simulink model "crazyflie"  (R2015b)
settings: Solver=FixedStepAuto  StartTime=0.0  StopTime=18  FixedStep=1/500  MinStep=1e-4  RelTol=1e-3
undefined symbols (not defined in the file): A, B, C, D
libraries: simulink x1
(part 2 of 3)

== system crazyflie/Off-board ILQR Position Controller/Subsystem2 ==
  Rollw : Inport
  Pitchw : Inport  Port=2
  Measured Yaw : Inport  Port=3
  Demux : Demux  Outputs=2
  MATLAB Function : MATLAB Function  TreatAsAtomicUnit=on
  Mux : Mux  Inputs=2
  Product : Product  Multiplication=Matrix(*)
  Rollb Error : Outport
  Pitchb Error : Outport  Port=2
  wires:
  Rollw/1 -> Mux/1
  Pitchw/1 -> Mux/2
  Product/1 -> Demux/1
  Demux/1 -> Rollb Error/1
  Demux/2 -> Pitchb Error/1
  Measured Yaw/1 -> MATLAB Function/1(yaw)
  MATLAB Function/1(R_m) -> Product/1
  Mux/1 -> Product/2  "Xw Error"

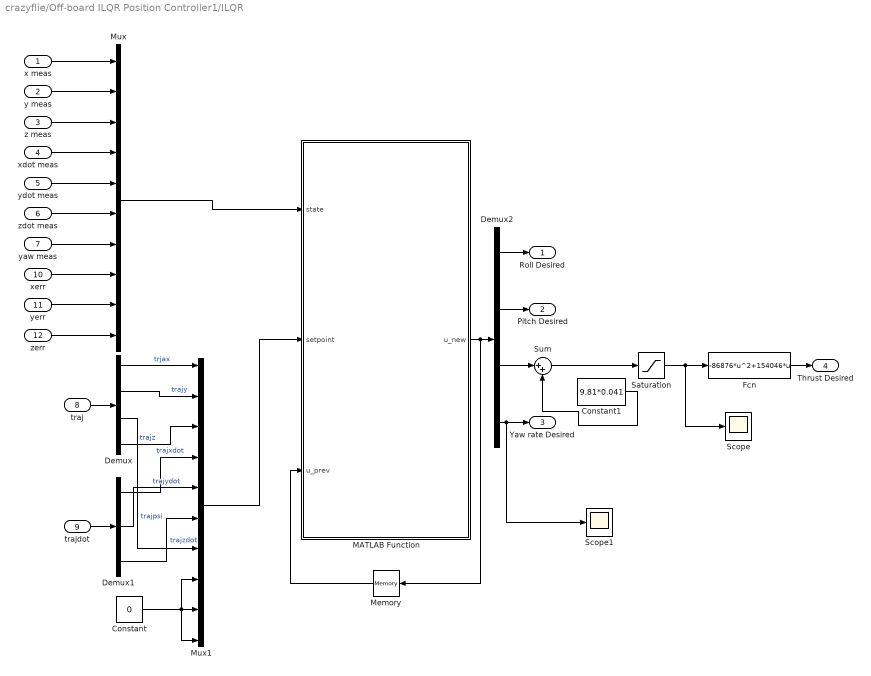
== system crazyflie/Off-board ILQR Position Controller1/ILQR ==
  x meas : Inport
  y meas : Inport  Port=2
  z meas : Inport  Port=3
  xdot meas : Inport  Port=4
  ydot meas : Inport  Port=5
  zdot meas : Inport  Port=6
  "yaw meas " : Inport  Port=7
  traj : Inport  Port=8
  trajdot : Inport  Port=9
  xerr : Inport  Port=10
  yerr : Inport  Port=11
  zerr : Inport  Port=12
  Constant : Constant  Value=0
  Constant1 : Constant  Value=9.81*0.041
  Demux : Demux
  Demux1 : Demux  Outputs=3
  Demux2 : Demux
  Fcn : Fcn  Expr=-86876*u^2+154046*u
  MATLAB Function : MATLAB Function  TreatAsAtomicUnit=on
  Memory : Memory  X0=[0 0 0 0]'
  Mux : Mux  Inputs=10
  Mux1 : Mux  Inputs=10
  Saturation : Saturate  UpperLimit=0.65  LowerLimit=0
  Scope : Scope
  Scope1 : Scope
  Sum : Sum  Inputs=|++
  Roll Desired : Outport
  Pitch Desired : Outport  Port=2
  Yaw rate Desired : Outport  Port=3
  Thrust Desired : Outport  Port=4
  wires:
  x meas/1 -> Mux/1
  y meas/1 -> Mux/2
  Fcn/1 -> Thrust Desired/1
  z meas/1 -> Mux/3
  ydot meas/1 -> Mux/5
  zdot meas/1 -> Mux/6
  "yaw meas "/1 -> Mux/7
  xdot meas/1 -> Mux/4
  Sum/1 -> Saturation/1
  Constant1/1 -> Sum/2
  traj/1 -> Demux/1
  trajdot/1 -> Demux1/1
  Mux/1 -> MATLAB Function/1(state)
  Mux1/1 -> MATLAB Function/2(setpoint)
  Demux/1 -> Mux1/1  "trjax"
  Demux/2 -> Mux1/2  "trajy"
  Demux/4 -> Mux1/3  "trajz"
  Demux1/1 -> Mux1/4  "trajxdot"
  Demux1/2 -> Mux1/5  "trajydot"
  Demux1/3 -> Mux1/6  "trajzdot"
  Demux/3 -> Mux1/7  "trajpsi"
  MATLAB Function/1(u_new) -> Demux2/1, Memory/1
  Memory/1 -> MATLAB Function/3(u_prev)
  Demux2/1 -> Roll Desired/1
  Demux2/2 -> Pitch Desired/1
  Demux2/4 -> Yaw rate Desired/1, Scope1/1
  Demux2/3 -> Sum/1
  Saturation/1 -> Scope/1, Fcn/1
  Constant/1 -> Mux1/10, Mux1/8, Mux1/9
  xerr/1 -> Mux/8
  yerr/1 -> Mux/9
  zerr/1 -> Mux/10

== system crazyflie/Off-board ILQR Position Controller1/Subsystem2 ==
  Rollw : Inport
  Pitchw : Inport  Port=2
  Measured Yaw : Inport  Port=3
  Demux : Demux  Outputs=2
  MATLAB Function : MATLAB Function  TreatAsAtomicUnit=on
  Mux : Mux  Inputs=2
  Product : Product  Multiplication=Matrix(*)
  Rollb Error : Outport
  Pitchb Error : Outport  Port=2
  wires:
  Rollw/1 -> Mux/1
  Pitchw/1 -> Mux/2
  Product/1 -> Demux/1
  Demux/1 -> Rollb Error/1
  Demux/2 -> Pitchb Error/1
  Measured Yaw/1 -> MATLAB Function/1(yaw)
  MATLAB Function/1(R_m) -> Product/1
  Mux/1 -> Product/2  "Xw Error"

== system crazyflie/Off-board LQR Position Controller /LQR ==
  xe : Inport
  ye : Inport  Port=2
  ze : Inport  Port=3
  xdote : Inport  Port=4
  ydote : Inport  Port=5
  zdote : Inport  Port=6
  "yawe " : Inport  Port=7
  xe int : Inport  Port=8
  ye int : Inport  Port=9
  ze int : Inport  Port=10
  Constant : Constant  Value="[5.60004970078151\t8.58620031779818e-15\t1.79188398034056e-13\t10.0569231021990\t1.51538658702357e-16\t6.75183288667297e-14\t-5.69346371635233e-16\t0.316227766016842\t1.15721882726472e-16\t7.37858743577978e-16;-4.45384218978841e-15\t5.60004970078150\t1.40244562919347e-12\t1.51538658702357e-16\t10.0569231021990\t2.52099816991567e-13\t-1.20831577789100e-16\t3.71448157568776e-15\t0.316227766016834\t6.21616501237700e-13;-1.24071227397705e-14\t1.04992513941598e-14\t316.738599971154\t1.66810943507647e-17\t6.22838406049332e-17\t511.246554592667\t-5.10238077464527e-16\t-2.21761716133426e-16\t9.39771534804335e-15\t0.316227766016796;-5.87842517815967e-15\t-1.61107236968454e-15\t-1.26223470684901e-13\t-5.80373467518077e-17\t-1.23171842802345e-17\t-2.10523704707751e-13\t3.16227766016838\t-1.11614612446732e-15\t2.11077368256129e-16\t-6.41049593874995e-15]"
  Constant1 : Constant  Value=9.81*0.041
  Demux : Demux
  Fcn : Fcn  Expr=-86876*u^2+154046*u
  Mux : Mux  Inputs=10
  Product : Product  Multiplication=Matrix(*)
  Saturation : Saturate  UpperLimit=0.65  LowerLimit=-0.041*9.81
  Sum : Sum  Inputs=|++
  Roll Desired : Outport
  Pitch Desired : Outport  Port=2
  Yaw rate Desired : Outport  Port=3
  Thrust Desired : Outport  Port=4
  wires:
  xe/1 -> Mux/1
  ye/1 -> Mux/2
  Demux/1 -> Roll Desired/1
  Demux/2 -> Pitch Desired/1
  Fcn/1 -> Thrust Desired/1
  ze/1 -> Mux/3
  ydote/1 -> Mux/5
  zdote/1 -> Mux/6
  Demux/3 -> Saturation/1
  Demux/4 -> Yaw rate Desired/1
  Mux/1 -> Product/2
  Product/1 -> Demux/1
  Constant/1 -> Product/1
  "yawe "/1 -> Mux/7
  xdote/1 -> Mux/4
  xe int/1 -> Mux/8
  ye int/1 -> Mux/9
  ze int/1 -> Mux/10
  Saturation/1 -> Sum/1
  Sum/1 -> Fcn/1
  Constant1/1 -> Sum/2

== system crazyflie/Off-board LQR Position Controller /Subsystem ==
  X : Inport
  Measured X : Inport  Port=2
  Y : Inport  Port=3
  Measured Y : Inport  Port=4
  Measured Yaw : Inport  Port=5
  Demux : Demux  Outputs=2
  MATLAB Function : MATLAB Function  TreatAsAtomicUnit=on
  Mux : Mux  Inputs=2
  Product : Product  Multiplication=Matrix(*)
  Sum : Sum  Inputs=|+-
  Sum1 : Sum  Inputs=|+-
  Xb Error : Outport
  Yb Error : Outport  Port=2
  wires:
  X/1 -> Sum/1
  Measured X/1 -> Sum/2
  Y/1 -> Sum1/1
  Measured Y/1 -> Sum1/2
  Sum/1 -> Mux/1
  Sum1/1 -> Mux/2
  Product/1 -> Demux/1
  Demux/1 -> Xb Error/1
  Demux/2 -> Yb Error/1
  Measured Yaw/1 -> MATLAB Function/1(yaw)
  MATLAB Function/1(R_m) -> Product/1
  Mux/1 -> Product/2  "Xw Error"

== system crazyflie/Off-board LQR Position Controller /Subsystem1 ==
  Xdot : Inport
  Measured Xdot : Inport  Port=2
  Ydot : Inport  Port=3
  Measured Ydot : Inport  Port=4
  Measured Yaw : Inport  Port=5
  Demux : Demux  Outputs=2
  MATLAB Function : MATLAB Function  TreatAsAtomicUnit=on
  Mux : Mux  Inputs=2
  Product : Product  Multiplication=Matrix(*)
  Sum : Sum  Inputs=|+-
  Sum1 : Sum  Inputs=|+-
  Xdotb Error : Outport
  Ydotb Error : Outport  Port=2
  wires:
  Xdot/1 -> Sum/1
  Measured Xdot/1 -> Sum/2
  Ydot/1 -> Sum1/1
  Measured Ydot/1 -> Sum1/2
  Sum/1 -> Mux/1
  Sum1/1 -> Mux/2
  Product/1 -> Demux/1
  Demux/1 -> Xdotb Error/1
  Demux/2 -> Ydotb Error/1
  Measured Yaw/1 -> MATLAB Function/1(yaw)
  MATLAB Function/1(R_m) -> Product/1
  Mux/1 -> Product/2  "Xw Error"

== system crazyflie/Off-board PID Position Controller/Subsystem ==
  X : Inport
  Measured X : Inport  Port=2
  Y : Inport  Port=3
  Measured Y : Inport  Port=4
  Measured Yaw : Inport  Port=5
  Demux : Demux  Outputs=2
  MATLAB Function : MATLAB Function  TreatAsAtomicUnit=on
  Mux : Mux  Inputs=2
  Product : Product  Multiplication=Matrix(*)
  Sum : Sum  Inputs=|+-
  Sum1 : Sum  Inputs=|+-
  Xb Error : Outport
  Yb Error : Outport  Port=2
  wires:
  X/1 -> Sum/1
  Measured X/1 -> Sum/2
  Y/1 -> Sum1/1
  Measured Y/1 -> Sum1/2
  Sum/1 -> Mux/1
  Sum1/1 -> Mux/2
  Product/1 -> Demux/1
  Demux/1 -> Xb Error/1
  Demux/2 -> Yb Error/1
  Measured Yaw/1 -> MATLAB Function/1(yaw)
  MATLAB Function/1(R_m) -> Product/1
  Mux/1 -> Product/2  "Xw Error"

== system crazyflie/Off-board PID Position Controller/X PID ==
  Xb Error : Inport
  Derivative : Derivative
  Integrator : Integrator
  Kd : Gain  Gain=10
  Ki : Gain  Gain=4
  Kp : Gain  Gain=18
  Saturation : Saturate  UpperLimit=.2  LowerLimit=-.2
  Sine Wave : Sin  Amplitude=0  SampleTime=0
  Sum : Sum  Inputs=|++
  Sum3 : Sum  Inputs=+++
  X PID : Outport
  wires:
  Xb Error/1 -> Derivative/1, Integrator/1, Kp/1
  Kp/1 -> Sum3/1
  Kd/1 -> Sum3/3
  Ki/1 -> Sum3/2
  Saturation/1 -> Ki/1
  Integrator/1 -> Saturation/1
  Derivative/1 -> Kd/1
  Sum/1 -> X PID/1
  Sine Wave/1 -> Sum/2
  Sum3/1 -> Sum/1

== system crazyflie/Off-board PID Position Controller/Y PID ==
  Yb Error : Inport
  Derivative : Derivative
  Integrator : Integrator
  Kd : Gain  Gain=10
  Ki : Gain  Gain=4
  Kp : Gain  Gain=18
  Saturation : Saturate  UpperLimit=.2  LowerLimit=-.2
  Sine Wave : Sin  Amplitude=0  SampleTime=0
  Sum : Sum  Inputs=|++
  Sum3 : Sum  Inputs=+++
  Y PID : Outport
  wires:
  Yb Error/1 -> Derivative/1, Integrator/1, Kp/1
  Kp/1 -> Sum3/1
  Kd/1 -> Sum3/3
  Ki/1 -> Sum3/2
  Saturation/1 -> Ki/1
  Integrator/1 -> Saturation/1
  Derivative/1 -> Kd/1
  Sum/1 -> Y PID/1
  Sine Wave/1 -> Sum/2
  Sum3/1 -> Sum/1

== system crazyflie/Off-board PID Position Controller/Yaw PID ==
  Yaw : Inport
  Measured Yaw : Inport  Port=2
  Derivative : Derivative
  Integrator : Integrator
  Kd : Gain
  Ki : Gain  Gain=0
  Kp : Gain  Gain=3
  Saturation : Saturate  UpperLimit=.2  LowerLimit=-.2
  Sine Wave : Sin  Amplitude=0  SampleTime=0
  Sum : Sum  Inputs=|++
  Sum2 : Sum  Inputs=|+-
  Sum3 : Sum  Inputs=+++
  Yaw PID : Outport
  wires:
  Yaw/1 -> Sum2/1
  Measured Yaw/1 -> Sum2/2
  Sum2/1 -> Derivative/1, Integrator/1, Kp/1
  Kp/1 -> Sum3/1
  Kd/1 -> Sum3/3
  Ki/1 -> Sum3/2
  Saturation/1 -> Ki/1
  Integrator/1 -> Saturation/1
  Derivative/1 -> Kd/1
  Sine Wave/1 -> Sum/2
  Sum3/1 -> Sum/1
  Sum/1 -> Yaw PID/1

== system crazyflie/Off-board PID Position Controller/Z PID ==
  Z : Inport
  Measured Z : Inport  Port=2
  Derivative : Derivative
  Integrator : Integrator
  Kd : Gain  Gain=40000
  Ki : Gain  Gain=10000
  Kp : Gain  Gain=50000
  PID Limit : Saturate  UpperLimit=25000  LowerLimit=-25000
  Saturation : Saturate  UpperLimit=10  LowerLimit=-10
  Sine Wave : Sin  Amplitude=0  SampleTime=0
  Sum : Sum  Inputs=|++
  Sum1 : Sum  Inputs=|++
  Sum2 : Sum  Inputs=|+-
  Sum3 : Sum  Inputs=+++
  Thrust Base : Constant  Value=36500
  Z PID : Outport
  wires:
  Sum2/1 -> Integrator/1, Derivative/1, Kp/1
  Kp/1 -> Sum3/1
  Kd/1 -> Sum3/3
  Ki/1 -> Sum3/2
  Saturation/1 -> Ki/1
  Thrust Base/1 -> Sum/2
  Sum3/1 -> PID Limit/1
  PID Limit/1 -> Sum/1
  Z/1 -> Sum2/1
  Measured Z/1 -> Sum2/2
  Integrator/1 -> Saturation/1
  Derivative/1 -> Kd/1
  Sum/1 -> Sum1/1
  Sum1/1 -> Z PID/1
  Sine Wave/1 -> Sum1/2

== system crazyflie/Off-board PID Position Controller1/Subsystem ==
  X : Inport
  Measured X : Inport  Port=2
  Y : Inport  Port=3
  Measured Y : Inport  Port=4
  Measured Yaw : Inport  Port=5
  Demux : Demux  Outputs=2
  MATLAB Function : MATLAB Function  TreatAsAtomicUnit=on
  Mux : Mux  Inputs=2
  Product : Product  Multiplication=Matrix(*)
  Sum : Sum  Inputs=|+-
  Sum1 : Sum  Inputs=|+-
  Xb Error : Outport
  Yb Error : Outport  Port=2
  wires:
  X/1 -> Sum/1
  Measured X/1 -> Sum/2
  Y/1 -> Sum1/1
  Measured Y/1 -> Sum1/2
  Sum/1 -> Mux/1
  Sum1/1 -> Mux/2
  Product/1 -> Demux/1
  Demux/1 -> Xb Error/1
  Demux/2 -> Yb Error/1
  Measured Yaw/1 -> MATLAB Function/1(yaw)
  MATLAB Function/1(R_m) -> Product/1
  Mux/1 -> Product/2  "Xw Error"

== system crazyflie/Off-board PID Position Controller1/X PID ==
  Xb Error : Inport
  Derivative : Derivative
  Integrator : Integrator
  Kd : Gain  Gain=10
  Ki : Gain  Gain=4
  Kp : Gain  Gain=18
  Saturation : Saturate  UpperLimit=.2  LowerLimit=-.2
  Sum3 : Sum  Inputs=+++
  X PID : Outport
  wires:
  Xb Error/1 -> Derivative/1, Integrator/1, Kp/1
  Kp/1 -> Sum3/1
  Kd/1 -> Sum3/3
  Sum3/1 -> X PID/1
  Ki/1 -> Sum3/2
  Saturation/1 -> Ki/1
  Integrator/1 -> Saturation/1
  Derivative/1 -> Kd/1

== system crazyflie/Off-board PID Position Controller1/Y PID ==
  Yb Error : Inport
  Derivative : Derivative
  Integrator : Integrator
  Kd : Gain  Gain=10
  Ki : Gain  Gain=4
  Kp : Gain  Gain=18
  Saturation : Saturate  UpperLimit=.2  LowerLimit=-.2
  Sum3 : Sum  Inputs=+++
  Y PID : Outport
  wires:
  Yb Error/1 -> Derivative/1, Integrator/1, Kp/1
  Kp/1 -> Sum3/1
  Kd/1 -> Sum3/3
  Sum3/1 -> Y PID/1
  Ki/1 -> Sum3/2
  Saturation/1 -> Ki/1
  Integrator/1 -> Saturation/1
  Derivative/1 -> Kd/1

== system crazyflie/Off-board PID Position Controller1/Yaw PID ==
  Yaw : Inport
  Measured Yaw : Inport  Port=2
  Derivative : Derivative
  Integrator : Integrator
  Kd : Gain
  Ki : Gain  Gain=0
  Kp : Gain  Gain=3
  Saturation : Saturate  UpperLimit=.2  LowerLimit=-.2
  Sum2 : Sum  Inputs=|+-
  Sum3 : Sum  Inputs=+++
  Yaw PID : Outport
  wires:
  Yaw/1 -> Sum2/1
  Measured Yaw/1 -> Sum2/2
  Sum2/1 -> Derivative/1, Integrator/1, Kp/1
  Kp/1 -> Sum3/1
  Kd/1 -> Sum3/3
  Sum3/1 -> Yaw PID/1
  Ki/1 -> Sum3/2
  Saturation/1 -> Ki/1
  Integrator/1 -> Saturation/1
  Derivative/1 -> Kd/1

== system crazyflie/Off-board PID Position Controller1/Z PID ==
  Z : Inport
  Measured Z : Inport  Port=2
  Derivative : Derivative
  Integrator : Integrator
  Kd : Gain  Gain=40000
  Ki : Gain  Gain=10000
  Kp : Gain  Gain=50000
  PID Limit : Saturate  UpperLimit=25000  LowerLimit=-25000
  Saturation : Saturate  UpperLimit=10  LowerLimit=-10
  Sum : Sum  Inputs=|++
  Sum2 : Sum  Inputs=|+-
  Sum3 : Sum  Inputs=+++
  Thrust Base : Constant  Value=35125.3
  Z PID : Outport
  wires:
  Sum2/1 -> Integrator/1, Derivative/1, Kp/1
  Kp/1 -> Sum3/1
  Kd/1 -> Sum3/3
  Ki/1 -> Sum3/2
  Saturation/1 -> Ki/1
  Thrust Base/1 -> Sum/2
  Sum/1 -> Z PID/1
  Sum3/1 -> PID Limit/1
  PID Limit/1 -> Sum/1
  Z/1 -> Sum2/1
  Measured Z/1 -> Sum2/2
  Integrator/1 -> Saturation/1
  Derivative/1 -> Kd/1

== system crazyflie/On-board Controller/Attitude Controller  ==
  Roll : Inport
  Pitch : Inport  Port=2
  Measured Roll : Inport  Port=3
  Measured Pitch : Inport  Port=4
  Pitch PID : Subsystem
  Roll PID : Subsystem
  Desired Roll : Outport
  "Desired Pitch " : Outport  Port=2
  wires:
  Pitch/1 -> Pitch PID/1(Pitch)
  Measured Pitch/1 -> Pitch PID/2(Measured Pitch)
  Pitch PID/1(Pitch PID) -> "Desired Pitch "/1
  Measured Roll/1 -> Roll PID/2(Measured Roll)
  Roll/1 -> Roll PID/1(Roll)
  Roll PID/1(Roll PID) -> Desired Roll/1

== system crazyflie/On-board Controller/Attitude Rate Controller ==
  Roll Rate : Inport
  Pitch Rate : Inport  Port=2
  Measured Roll Rate : Inport  Port=3
  Measured Pitch Rate : Inport  Port=4
  Pitch Rate PID : Subsystem
  Roll Rate PID : Subsystem
  Saturation : Saturate  UpperLimit=2^15  LowerLimit=-2^15
  Saturation1 : Saturate  UpperLimit=2^15  LowerLimit=-2^15
  Commanded Roll : Outport
  Commanded Pitch : Outport  Port=2
  wires:
  Roll Rate/1 -> Roll Rate PID/1(Roll Rate)
  Measured Roll Rate/1 -> Roll Rate PID/2(Measured Roll Rate)
  Pitch Rate/1 -> Pitch Rate PID/1(Pitch Ratel)
  Measured Pitch Rate/1 -> Pitch Rate PID/2(Measured Pitch Rate)
  Roll Rate PID/1(Roll Rate PID) -> Saturation/1
  Pitch Rate PID/1(Pitch Rate PID) -> Saturation1/1
  Saturation/1 -> Commanded Roll/1
  Saturation1/1 -> Commanded Pitch/1

== system crazyflie/On-board Controller/Mixer ==
  Roll : Inport
  Pitch : Inport  Port=2
  Yawrate : Inport  Port=3
  Thrust : Inport  Port=4
  Display : Display
  Gain : Gain  Gain=.5
  Gain1 : Gain  Gain=.5
  Saturation{,1..3} (4 alike) : Saturate  UpperLimit=2^16  LowerLimit=0
  Sum : Sum  Inputs=-+++
  Sum1 : Sum  Inputs=---+
  Sum2 : Sum  Inputs=+-++
  Sum3 : Sum  Inputs=++-+
  Motor 1 : Outport
  Motor 2 : Outport  Port=2
  Motor 3 : Outport  Port=3
  Motor 4 : Outport  Port=4
  wires:
  Roll/1 -> Gain/1
  Pitch/1 -> Gain1/1
  Yawrate/1 -> Sum1/3, Sum/3, Sum3/3, Sum2/3
  Thrust/1 -> Sum2/4, Sum3/4, Sum1/4, Sum/4
  Sum/1 -> Saturation/1
  Sum2/1 -> Saturation2/1
  Sum3/1 -> Saturation3/1
  Sum1/1 -> Saturation1/1
  Gain/1 -> Sum3/1, Sum2/1, Sum1/1, Sum/1
  Gain1/1 -> Sum3/2, Sum2/2, Sum1/2, Sum/2
  Saturation1/1 -> Motor 2/1
  Saturation2/1 -> Motor 3/1
  Saturation3/1 -> Motor 4/1
  Saturation/1 -> Display/1, Motor 1/1

== system crazyflie/On-board Controller/Yawrate Controller  ==
  Desired Yawrate : Inport
  Measured Yawrate : Inport  Port=2
  Yawrate PID : Subsystem
  Commanded Yawrate : Outport
  wires:
  Yawrate PID/1(Yawrate PID) -> Commanded Yawrate/1
  Desired Yawrate/1 -> Yawrate PID/1(Yawrate)
  Measured Yawrate/1 -> Yawrate PID/2(Measured Yawrate)

== system crazyflie/On-board Controller1/Attitude Controller  ==
  Roll : Inport
  Pitch : Inport  Port=2
  Measured Roll : Inport  Port=3
  Measured Pitch : Inport  Port=4
  Pitch PID : Subsystem
  Roll PID : Subsystem
  Desired Roll : Outport
  "Desired Pitch " : Outport  Port=2
  wires:
  Pitch/1 -> Pitch PID/1(Pitch)
  Measured Pitch/1 -> Pitch PID/2(Measured Pitch)
  Pitch PID/1(Pitch PID) -> "Desired Pitch "/1
  Measured Roll/1 -> Roll PID/2(Measured Roll)
  Roll/1 -> Roll PID/1(Roll)
  Roll PID/1(Roll PID) -> Desired Roll/1

== system crazyflie/On-board Controller1/Attitude Rate Controller ==
  Roll Rate : Inport
  Pitch Rate : Inport  Port=2
  Measured Roll Rate : Inport  Port=3
  Measured Pitch Rate : Inport  Port=4
  Pitch Rate PID : Subsystem
  Roll Rate PID : Subsystem
  Saturation : Saturate  UpperLimit=2^15  LowerLimit=-2^15
  Saturation1 : Saturate  UpperLimit=2^15  LowerLimit=-2^15
  Commanded Roll : Outport
  Commanded Pitch : Outport  Port=2
  wires:
  Roll Rate/1 -> Roll Rate PID/1(Roll Rate)
  Measured Roll Rate/1 -> Roll Rate PID/2(Measured Roll Rate)
  Pitch Rate/1 -> Pitch Rate PID/1(Pitch Ratel)
  Measured Pitch Rate/1 -> Pitch Rate PID/2(Measured Pitch Rate)
  Roll Rate PID/1(Roll Rate PID) -> Saturation/1
  Pitch Rate PID/1(Pitch Rate PID) -> Saturation1/1
  Saturation/1 -> Commanded Roll/1
  Saturation1/1 -> Commanded Pitch/1

== system crazyflie/On-board Controller1/Mixer ==
  Roll : Inport
  Pitch : Inport  Port=2
  Yawrate : Inport  Port=3
  Thrust : Inport  Port=4
  Display : Display
  Gain : Gain  Gain=.5
  Gain1 : Gain  Gain=.5
  Saturation{,1..3} (4 alike) : Saturate  UpperLimit=2^16  LowerLimit=0
  Sum : Sum  Inputs=-+++
  Sum1 : Sum  Inputs=---+
  Sum2 : Sum  Inputs=+-++
  Sum3 : Sum  Inputs=++-+
  Motor 1 : Outport
  Motor 2 : Outport  Port=2
  Motor 3 : Outport  Port=3
  Motor 4 : Outport  Port=4
  wires:
  Roll/1 -> Gain/1
  Pitch/1 -> Gain1/1
  Yawrate/1 -> Sum1/3, Sum/3, Sum3/3, Sum2/3
  Thrust/1 -> Sum2/4, Sum3/4, Sum1/4, Sum/4
  Sum/1 -> Saturation/1
  Sum2/1 -> Saturation2/1
  Sum3/1 -> Saturation3/1
  Sum1/1 -> Saturation1/1
  Gain/1 -> Sum3/1, Sum2/1, Sum1/1, Sum/1
  Gain1/1 -> Sum3/2, Sum2/2, Sum1/2, Sum/2
  Saturation1/1 -> Motor 2/1
  Saturation2/1 -> Motor 3/1
  Saturation3/1 -> Motor 4/1
  Saturation/1 -> Display/1, Motor 1/1

== system crazyflie/On-board Controller1/Yawrate Controller  ==
  Desired Yawrate : Inport
  Measured Yawrate : Inport  Port=2
  Yawrate PID : Subsystem
  Commanded Yawrate : Outport
  wires:
  Yawrate PID/1(Yawrate PID) -> Commanded Yawrate/1
  Desired Yawrate/1 -> Yawrate PID/1(Yawrate)
  Measured Yawrate/1 -> Yawrate PID/2(Measured Yawrate)

== system crazyflie/On-board Controller2/Attitude Controller  ==
  Roll : Inport
  Pitch : Inport  Port=2
  Measured Roll : Inport  Port=3
  Measured Pitch : Inport  Port=4
  Pitch PID : Subsystem
  Roll PID : Subsystem
  Desired Roll : Outport
  "Desired Pitch " : Outport  Port=2
  wires:
  Pitch/1 -> Pitch PID/1(Pitch)
  Measured Pitch/1 -> Pitch PID/2(Measured Pitch)
  Pitch PID/1(Pitch PID) -> "Desired Pitch "/1
  Measured Roll/1 -> Roll PID/2(Measured Roll)
  Roll/1 -> Roll PID/1(Roll)
  Roll PID/1(Roll PID) -> Desired Roll/1

== system crazyflie/On-board Controller2/Attitude Rate Controller ==
  Roll Rate : Inport
  Pitch Rate : Inport  Port=2
  Measured Roll Rate : Inport  Port=3
  Measured Pitch Rate : Inport  Port=4
  Pitch Rate PID : Subsystem
  Roll Rate PID : Subsystem
  Saturation : Saturate  UpperLimit=2^15  LowerLimit=-2^15
  Saturation1 : Saturate  UpperLimit=2^15  LowerLimit=-2^15
  Commanded Roll : Outport
  Commanded Pitch : Outport  Port=2
  wires:
  Roll Rate/1 -> Roll Rate PID/1(Roll Rate)
  Measured Roll Rate/1 -> Roll Rate PID/2(Measured Roll Rate)
  Pitch Rate/1 -> Pitch Rate PID/1(Pitch Ratel)
  Measured Pitch Rate/1 -> Pitch Rate PID/2(Measured Pitch Rate)
  Roll Rate PID/1(Roll Rate PID) -> Saturation/1
  Pitch Rate PID/1(Pitch Rate PID) -> Saturation1/1
  Saturation/1 -> Commanded Roll/1
  Saturation1/1 -> Commanded Pitch/1

== system crazyflie/On-board Controller2/Mixer ==
  Roll : Inport
  Pitch : Inport  Port=2
  Yawrate : Inport  Port=3
  Thrust : Inport  Port=4
  Display : Display
  Gain : Gain  Gain=.5
  Gain1 : Gain  Gain=.5
  Saturation{,1..3} (4 alike) : Saturate  UpperLimit=2^16  LowerLimit=0
  Sum : Sum  Inputs=-+++
  Sum1 : Sum  Inputs=---+
  Sum2 : Sum  Inputs=+-++
  Sum3 : Sum  Inputs=++-+
  Motor 1 : Outport
  Motor 2 : Outport  Port=2
  Motor 3 : Outport  Port=3
  Motor 4 : Outport  Port=4
  wires:
  Roll/1 -> Gain/1
  Pitch/1 -> Gain1/1
  Yawrate/1 -> Sum1/3, Sum/3, Sum3/3, Sum2/3
  Thrust/1 -> Sum2/4, Sum3/4, Sum1/4, Sum/4
  Sum/1 -> Saturation/1
  Sum2/1 -> Saturation2/1
  Sum3/1 -> Saturation3/1
  Sum1/1 -> Saturation1/1
  Gain/1 -> Sum3/1, Sum2/1, Sum1/1, Sum/1
  Gain1/1 -> Sum3/2, Sum2/2, Sum1/2, Sum/2
  Saturation1/1 -> Motor 2/1
  Saturation2/1 -> Motor 3/1
  Saturation3/1 -> Motor 4/1
  Saturation/1 -> Display/1, Motor 1/1

== system crazyflie/On-board Controller2/Yawrate Controller  ==
  Desired Yawrate : Inport
  Measured Yawrate : Inport  Port=2
  Yawrate PID : Subsystem
  Commanded Yawrate : Outport
  wires:
  Yawrate PID/1(Yawrate PID) -> Commanded Yawrate/1
  Desired Yawrate/1 -> Yawrate PID/1(Yawrate)
  Measured Yawrate/1 -> Yawrate PID/2(Measured Yawrate)

== system crazyflie/On-board Controller3/Attitude Controller  ==
  Roll : Inport
  Pitch : Inport  Port=2
  Measured Roll : Inport  Port=3
  Measured Pitch : Inport  Port=4
  Pitch PID : Subsystem
  Roll PID : Subsystem
  Desired Roll : Outport
  "Desired Pitch " : Outport  Port=2
  wires:
  Pitch/1 -> Pitch PID/1(Pitch)
  Measured Pitch/1 -> Pitch PID/2(Measured Pitch)
  Pitch PID/1(Pitch PID) -> "Desired Pitch "/1
  Measured Roll/1 -> Roll PID/2(Measured Roll)
  Roll/1 -> Roll PID/1(Roll)
  Roll PID/1(Roll PID) -> Desired Roll/1

== system crazyflie/On-board Controller3/Attitude Rate Controller ==
  Roll Rate : Inport
  Pitch Rate : Inport  Port=2
  Measured Roll Rate : Inport  Port=3
  Measured Pitch Rate : Inport  Port=4
  Pitch Rate PID : Subsystem
  Roll Rate PID : Subsystem
  Saturation : Saturate  UpperLimit=2^15  LowerLimit=-2^15
  Saturation1 : Saturate  UpperLimit=2^15  LowerLimit=-2^15
  Commanded Roll : Outport
  Commanded Pitch : Outport  Port=2
  wires:
  Roll Rate/1 -> Roll Rate PID/1(Roll Rate)
  Measured Roll Rate/1 -> Roll Rate PID/2(Measured Roll Rate)
  Pitch Rate/1 -> Pitch Rate PID/1(Pitch Ratel)
  Measured Pitch Rate/1 -> Pitch Rate PID/2(Measured Pitch Rate)
  Roll Rate PID/1(Roll Rate PID) -> Saturation/1
  Pitch Rate PID/1(Pitch Rate PID) -> Saturation1/1
  Saturation/1 -> Commanded Roll/1
  Saturation1/1 -> Commanded Pitch/1

== system crazyflie/On-board Controller3/Mixer ==
  Roll : Inport
  Pitch : Inport  Port=2
  Yawrate : Inport  Port=3
  Thrust : Inport  Port=4
  Display : Display
  Gain : Gain  Gain=.5
  Gain1 : Gain  Gain=.5
  Saturation{,1..3} (4 alike) : Saturate  UpperLimit=2^16  LowerLimit=0
  Sum : Sum  Inputs=-+++
  Sum1 : Sum  Inputs=---+
  Sum2 : Sum  Inputs=+-++
  Sum3 : Sum  Inputs=++-+
  Motor 1 : Outport
  Motor 2 : Outport  Port=2
  Motor 3 : Outport  Port=3
  Motor 4 : Outport  Port=4
  wires:
  Roll/1 -> Gain/1
  Pitch/1 -> Gain1/1
  Yawrate/1 -> Sum1/3, Sum/3, Sum3/3, Sum2/3
  Thrust/1 -> Sum2/4, Sum3/4, Sum1/4, Sum/4
  Sum/1 -> Saturation/1
  Sum2/1 -> Saturation2/1
  Sum3/1 -> Saturation3/1
  Sum1/1 -> Saturation1/1
  Gain/1 -> Sum3/1, Sum2/1, Sum1/1, Sum/1
  Gain1/1 -> Sum3/2, Sum2/2, Sum1/2, Sum/2
  Saturation1/1 -> Motor 2/1
  Saturation2/1 -> Motor 3/1
  Saturation3/1 -> Motor 4/1
  Saturation/1 -> Display/1, Motor 1/1

== system crazyflie/On-board Controller3/Yawrate Controller  ==
  Desired Yawrate : Inport
  Measured Yawrate : Inport  Port=2
  Yawrate PID : Subsystem
  Commanded Yawrate : Outport
  wires:
  Yawrate PID/1(Yawrate PID) -> Commanded Yawrate/1
  Desired Yawrate/1 -> Yawrate PID/1(Yawrate)
  Measured Yawrate/1 -> Yawrate PID/2(Measured Yawrate)

== system crazyflie/On-board Controller4/Attitude Controller  ==
  Roll : Inport
  Pitch : Inport  Port=2
  Measured Roll : Inport  Port=3
  Measured Pitch : Inport  Port=4
  Pitch PID : Subsystem
  Roll PID : Subsystem
  Desired Roll : Outport
  "Desired Pitch " : Outport  Port=2
  wires:
  Pitch/1 -> Pitch PID/1(Pitch)
  Measured Pitch/1 -> Pitch PID/2(Measured Pitch)
  Pitch PID/1(Pitch PID) -> "Desired Pitch "/1
  Measured Roll/1 -> Roll PID/2(Measured Roll)
  Roll/1 -> Roll PID/1(Roll)
  Roll PID/1(Roll PID) -> Desired Roll/1

== system crazyflie/On-board Controller4/Attitude Rate Controller ==
  Roll Rate : Inport
  Pitch Rate : Inport  Port=2
  Measured Roll Rate : Inport  Port=3
  Measured Pitch Rate : Inport  Port=4
  Pitch Rate PID : Subsystem
  Roll Rate PID : Subsystem
  Saturation : Saturate  UpperLimit=2^15  LowerLimit=-2^15
  Saturation1 : Saturate  UpperLimit=2^15  LowerLimit=-2^15
  Commanded Roll : Outport
  Commanded Pitch : Outport  Port=2
  wires:
  Roll Rate/1 -> Roll Rate PID/1(Roll Rate)
  Measured Roll Rate/1 -> Roll Rate PID/2(Measured Roll Rate)
  Pitch Rate/1 -> Pitch Rate PID/1(Pitch Ratel)
  Measured Pitch Rate/1 -> Pitch Rate PID/2(Measured Pitch Rate)
  Roll Rate PID/1(Roll Rate PID) -> Saturation/1
  Pitch Rate PID/1(Pitch Rate PID) -> Saturation1/1
  Saturation/1 -> Commanded Roll/1
  Saturation1/1 -> Commanded Pitch/1

== system crazyflie/On-board Controller4/Mixer ==
  Roll : Inport
  Pitch : Inport  Port=2
  Yawrate : Inport  Port=3
  Thrust : Inport  Port=4
  Display : Display
  Gain : Gain  Gain=.5
  Gain1 : Gain  Gain=.5
  Saturation{,1..3} (4 alike) : Saturate  UpperLimit=2^16  LowerLimit=0
  Sum : Sum  Inputs=-+++
  Sum1 : Sum  Inputs=---+
  Sum2 : Sum  Inputs=+-++
  Sum3 : Sum  Inputs=++-+
  Motor 1 : Outport
  Motor 2 : Outport  Port=2
  Motor 3 : Outport  Port=3
  Motor 4 : Outport  Port=4
  wires:
  Roll/1 -> Gain/1
  Pitch/1 -> Gain1/1
  Yawrate/1 -> Sum1/3, Sum/3, Sum3/3, Sum2/3
  Thrust/1 -> Sum2/4, Sum3/4, Sum1/4, Sum/4
  Sum/1 -> Saturation/1
  Sum2/1 -> Saturation2/1
  Sum3/1 -> Saturation3/1
  Sum1/1 -> Saturation1/1
  Gain/1 -> Sum3/1, Sum2/1, Sum1/1, Sum/1
  Gain1/1 -> Sum3/2, Sum2/2, Sum1/2, Sum/2
  Saturation1/1 -> Motor 2/1
  Saturation2/1 -> Motor 3/1
  Saturation3/1 -> Motor 4/1
  Saturation/1 -> Display/1, Motor 1/1

== system crazyflie/On-board Controller4/Yawrate Controller  ==
  Desired Yawrate : Inport
  Measured Yawrate : Inport  Port=2
  Yawrate PID : Subsystem
  Commanded Yawrate : Outport
  wires:
  Yawrate PID/1(Yawrate PID) -> Commanded Yawrate/1
  Desired Yawrate/1 -> Yawrate PID/1(Yawrate)
  Measured Yawrate/1 -> Yawrate PID/2(Measured Yawrate)

== system crazyflie/On-board Controller/Attitude Controller /Pitch PID ==
  Pitch : Inport
  Measured Pitch : Inport  Port=2
  Derivative : Derivative
  Integrator Limited : Integrator  LimitOutput=on  UpperSaturationLimit=20  LowerSaturationLimit=-20
  Kd1 : Gain  Gain=0
  Ki1 : Gain  Gain=4
  Kp1 : Gain  Gain=10
  Sum1 : Sum  Inputs=|+-
  Sum6 : Sum  Inputs=+++
  Pitch PID : Outport
  wires:
  Pitch/1 -> Sum1/1
  Measured Pitch/1 -> Sum1/2
  Sum1/1 -> Integrator Limited/1, Derivative/1, Kp1/1
  Kp1/1 -> Sum6/1
  Kd1/1 -> Sum6/3
  Sum6/1 -> Pitch PID/1
  Ki1/1 -> Sum6/2
  Derivative/1 -> Kd1/1
  Integrator Limited/1 -> Ki1/1

== system crazyflie/On-board Controller/Attitude Controller /Roll PID ==
  Roll : Inport
  Measured Roll : Inport  Port=2
  Derivative : Derivative
  Integrator Limited : Integrator  LimitOutput=on  UpperSaturationLimit=20  LowerSaturationLimit=-20
  Kd : Gain  Gain=0
  Ki : Gain  Gain=4
  Kp : Gain  Gain=10
  Sum2 : Sum  Inputs=|+-
  Sum3 : Sum  Inputs=+++
  Roll PID : Outport
  wires:
  Roll/1 -> Sum2/1
  Measured Roll/1 -> Sum2/2
  Sum2/1 -> Integrator Limited/1, Derivative/1, Kp/1
  Kp/1 -> Sum3/1
  Kd/1 -> Sum3/3
  Sum3/1 -> Roll PID/1
  Ki/1 -> Sum3/2
  Derivative/1 -> Kd/1
  Integrator Limited/1 -> Ki/1

== system crazyflie/On-board Controller/Attitude Rate Controller/Pitch Rate PID ==
  Pitch Ratel : Inport
  Measured Pitch Rate : Inport  Port=2
  Derivative : Derivative
  Integrator Limited : Integrator  LimitOutput=on  UpperSaturationLimit=33.3  LowerSaturationLimit=-33.3
  Kd : Gain  Gain=3
  Ki : Gain  Gain=550
  Kp : Gain  Gain=275
  Sum2 : Sum  Inputs=|+-
  Sum3 : Sum  Inputs=+++
  Pitch Rate PID : Outport
  wires:
  Pitch Ratel/1 -> Sum2/1
  Measured Pitch Rate/1 -> Sum2/2
  Sum2/1 -> Integrator Limited/1, Derivative/1, Kp/1
  Kp/1 -> Sum3/1
  Kd/1 -> Sum3/3
  Sum3/1 -> Pitch Rate PID/1
  Ki/1 -> Sum3/2
  Integrator Limited/1 -> Ki/1
  Derivative/1 -> Kd/1

== system crazyflie/On-board Controller/Attitude Rate Controller/Roll Rate PID ==
  Roll Rate : Inport
  Measured Roll Rate : Inport  Port=2
  Derivative : Derivative
  Integrator : Integrator
  Kd : Gain  Gain=3
  Ki : Gain  Gain=550
  Kp : Gain  Gain=275
  Saturation : Saturate  UpperLimit=33.3  LowerLimit=-33.3
  Sum2 : Sum  Inputs=|+-
  Sum3 : Sum  Inputs=+++
  Roll Rate PID : Outport
  wires:
  Roll Rate/1 -> Sum2/1
  Measured Roll Rate/1 -> Sum2/2
  Sum2/1 -> Derivative/1, Integrator/1, Kp/1
  Kp/1 -> Sum3/1
  Kd/1 -> Sum3/3
  Sum3/1 -> Roll Rate PID/1
  Ki/1 -> Sum3/2
  Saturation/1 -> Ki/1
  Integrator/1 -> Saturation/1
  Derivative/1 -> Kd/1

== system crazyflie/On-board Controller/Yawrate Controller /Yawrate PID ==
  Yawrate : Inport
  Measured Yawrate : Inport  Port=2
  Derivative : Derivative
  Integrator : Integrator
  Kd : Gain  Gain=0
  Ki : Gain  Gain=16.7
  Kp : Gain  Gain=70
  Saturation : Saturate  UpperLimit=166.7  LowerLimit=-166.7
  Sum : Sum  Inputs=|+-
  Sum1 : Sum  Inputs=+++
  Yawrate PID : Outport
  wires:
  Yawrate/1 -> Sum/1
  Measured Yawrate/1 -> Sum/2
  Sum/1 -> Integrator/1, Derivative/1, Kp/1
  Kp/1 -> Sum1/1
  Kd/1 -> Sum1/3
  Sum1/1 -> Yawrate PID/1
  Ki/1 -> Sum1/2
  Saturation/1 -> Ki/1
  Derivative/1 -> Kd/1
  Integrator/1 -> Saturation/1

== system crazyflie/On-board Controller1/Attitude Controller /Pitch PID ==
  Pitch : Inport
  Measured Pitch : Inport  Port=2
  Derivative : Derivative
  Integrator Limited : Integrator  LimitOutput=on  UpperSaturationLimit=20  LowerSaturationLimit=-20
  Kd1 : Gain  Gain=0
  Ki1 : Gain  Gain=4
  Kp1 : Gain  Gain=10
  Sum1 : Sum  Inputs=|+-
  Sum6 : Sum  Inputs=+++
  Pitch PID : Outport
  wires:
  Pitch/1 -> Sum1/1
  Measured Pitch/1 -> Sum1/2
  Sum1/1 -> Integrator Limited/1, Derivative/1, Kp1/1
  Kp1/1 -> Sum6/1
  Kd1/1 -> Sum6/3
  Sum6/1 -> Pitch PID/1
  Ki1/1 -> Sum6/2
  Derivative/1 -> Kd1/1
  Integrator Limited/1 -> Ki1/1

== system crazyflie/On-board Controller1/Attitude Controller /Roll PID ==
  Roll : Inport
  Measured Roll : Inport  Port=2
  Derivative : Derivative
  Integrator Limited : Integrator  LimitOutput=on  UpperSaturationLimit=20  LowerSaturationLimit=-20
  Kd : Gain  Gain=0
  Ki : Gain  Gain=4
  Kp : Gain  Gain=10
  Sum2 : Sum  Inputs=|+-
  Sum3 : Sum  Inputs=+++
  Roll PID : Outport
  wires:
  Roll/1 -> Sum2/1
  Measured Roll/1 -> Sum2/2
  Sum2/1 -> Integrator Limited/1, Derivative/1, Kp/1
  Kp/1 -> Sum3/1
  Kd/1 -> Sum3/3
  Sum3/1 -> Roll PID/1
  Ki/1 -> Sum3/2
  Derivative/1 -> Kd/1
  Integrator Limited/1 -> Ki/1

== system crazyflie/On-board Controller1/Attitude Rate Controller/Pitch Rate PID ==
  Pitch Ratel : Inport
  Measured Pitch Rate : Inport  Port=2
  Derivative : Derivative
  Integrator Limited : Integrator  LimitOutput=on  UpperSaturationLimit=33.3  LowerSaturationLimit=-33.3
  Kd : Gain  Gain=2.5
  Ki : Gain  Gain=500
  Kp : Gain  Gain=250
  Sum2 : Sum  Inputs=|+-
  Sum3 : Sum  Inputs=+++
  Pitch Rate PID : Outport
  wires:
  Pitch Ratel/1 -> Sum2/1
  Measured Pitch Rate/1 -> Sum2/2
  Sum2/1 -> Integrator Limited/1, Derivative/1, Kp/1
  Kp/1 -> Sum3/1
  Kd/1 -> Sum3/3
  Sum3/1 -> Pitch Rate PID/1
  Ki/1 -> Sum3/2
  Integrator Limited/1 -> Ki/1
  Derivative/1 -> Kd/1

== system crazyflie/On-board Controller1/Attitude Rate Controller/Roll Rate PID ==
  Roll Rate : Inport
  Measured Roll Rate : Inport  Port=2
  Derivative : Derivative
  Integrator : Integrator
  Kd : Gain  Gain=2.5
  Ki : Gain  Gain=500
  Kp : Gain  Gain=250
  Saturation : Saturate  UpperLimit=33.3  LowerLimit=-33.3
  Sum2 : Sum  Inputs=|+-
  Sum3 : Sum  Inputs=+++
  Roll Rate PID : Outport
  wires:
  Roll Rate/1 -> Sum2/1
  Measured Roll Rate/1 -> Sum2/2
  Sum2/1 -> Derivative/1, Integrator/1, Kp/1
  Kp/1 -> Sum3/1
  Kd/1 -> Sum3/3
  Sum3/1 -> Roll Rate PID/1
  Ki/1 -> Sum3/2
  Saturation/1 -> Ki/1
  Integrator/1 -> Saturation/1
  Derivative/1 -> Kd/1

== system crazyflie/On-board Controller1/Yawrate Controller /Yawrate PID ==
  Yawrate : Inport
  Measured Yawrate : Inport  Port=2
  Derivative : Derivative
  Integrator : Integrator
  Kd : Gain  Gain=0
  Ki : Gain  Gain=16.7
  Kp : Gain  Gain=70
  Saturation : Saturate  UpperLimit=166.7  LowerLimit=-166.7
  Sum : Sum  Inputs=|+-
  Sum1 : Sum  Inputs=+++
  Yawrate PID : Outport
  wires:
  Yawrate/1 -> Sum/1
  Measured Yawrate/1 -> Sum/2
  Sum/1 -> Integrator/1, Derivative/1, Kp/1
  Kp/1 -> Sum1/1
  Kd/1 -> Sum1/3
  Sum1/1 -> Yawrate PID/1
  Ki/1 -> Sum1/2
  Saturation/1 -> Ki/1
  Derivative/1 -> Kd/1
  Integrator/1 -> Saturation/1

== system crazyflie/On-board Controller2/Attitude Controller /Pitch PID ==
  Pitch : Inport
  Measured Pitch : Inport  Port=2
  Derivative : Derivative
  Integrator Limited : Integrator  LimitOutput=on  UpperSaturationLimit=20  LowerSaturationLimit=-20
  Kd1 : Gain  Gain=0
  Ki1 : Gain  Gain=4
  Kp1 : Gain  Gain=10
  Sum1 : Sum  Inputs=|+-
  Sum6 : Sum  Inputs=+++
  Pitch PID : Outport
  wires:
  Pitch/1 -> Sum1/1
  Measured Pitch/1 -> Sum1/2
  Sum1/1 -> Integrator Limited/1, Derivative/1, Kp1/1
  Kp1/1 -> Sum6/1
  Kd1/1 -> Sum6/3
  Sum6/1 -> Pitch PID/1
  Ki1/1 -> Sum6/2
  Derivative/1 -> Kd1/1
  Integrator Limited/1 -> Ki1/1

== system crazyflie/On-board Controller2/Attitude Controller /Roll PID ==
  Roll : Inport
  Measured Roll : Inport  Port=2
  Derivative : Derivative
  Integrator Limited : Integrator  LimitOutput=on  UpperSaturationLimit=20  LowerSaturationLimit=-20
  Kd : Gain  Gain=0
  Ki : Gain  Gain=4
  Kp : Gain  Gain=10
  Sum2 : Sum  Inputs=|+-
  Sum3 : Sum  Inputs=+++
  Roll PID : Outport
  wires:
  Roll/1 -> Sum2/1
  Measured Roll/1 -> Sum2/2
  Sum2/1 -> Integrator Limited/1, Derivative/1, Kp/1
  Kp/1 -> Sum3/1
  Kd/1 -> Sum3/3
  Sum3/1 -> Roll PID/1
  Ki/1 -> Sum3/2
  Derivative/1 -> Kd/1
  Integrator Limited/1 -> Ki/1

== system crazyflie/On-board Controller2/Attitude Rate Controller/Pitch Rate PID ==
  Pitch Ratel : Inport
  Measured Pitch Rate : Inport  Port=2
  Derivative : Derivative
  Integrator Limited : Integrator  LimitOutput=on  UpperSaturationLimit=33.3  LowerSaturationLimit=-33.3
  Kd : Gain  Gain=3
  Ki : Gain  Gain=550
  Kp : Gain  Gain=275
  Sum2 : Sum  Inputs=|+-
  Sum3 : Sum  Inputs=+++
  Pitch Rate PID : Outport
  wires:
  Pitch Ratel/1 -> Sum2/1
  Measured Pitch Rate/1 -> Sum2/2
  Sum2/1 -> Integrator Limited/1, Derivative/1, Kp/1
  Kp/1 -> Sum3/1
  Kd/1 -> Sum3/3
  Sum3/1 -> Pitch Rate PID/1
  Ki/1 -> Sum3/2
  Integrator Limited/1 -> Ki/1
  Derivative/1 -> Kd/1

== system crazyflie/On-board Controller2/Attitude Rate Controller/Roll Rate PID ==
  Roll Rate : Inport
  Measured Roll Rate : Inport  Port=2
  Derivative : Derivative
  Integrator : Integrator
  Kd : Gain  Gain=3
  Ki : Gain  Gain=550
  Kp : Gain  Gain=275
  Saturation : Saturate  UpperLimit=33.3  LowerLimit=-33.3
  Sum2 : Sum  Inputs=|+-
  Sum3 : Sum  Inputs=+++
  Roll Rate PID : Outport
  wires:
  Roll Rate/1 -> Sum2/1
  Measured Roll Rate/1 -> Sum2/2
  Sum2/1 -> Derivative/1, Integrator/1, Kp/1
  Kp/1 -> Sum3/1
  Kd/1 -> Sum3/3
  Sum3/1 -> Roll Rate PID/1
  Ki/1 -> Sum3/2
  Saturation/1 -> Ki/1
  Integrator/1 -> Saturation/1
  Derivative/1 -> Kd/1

== system crazyflie/On-board Controller2/Yawrate Controller /Yawrate PID ==
  Yawrate : Inport
  Measured Yawrate : Inport  Port=2
  Derivative : Derivative
  Integrator : Integrator
  Kd : Gain  Gain=0
  Ki : Gain  Gain=16.7
  Kp : Gain  Gain=70
  Saturation : Saturate  UpperLimit=166.7  LowerLimit=-166.7
  Sum : Sum  Inputs=|+-
  Sum1 : Sum  Inputs=+++
  Yawrate PID : Outport
  wires:
  Yawrate/1 -> Sum/1
  Measured Yawrate/1 -> Sum/2
  Sum/1 -> Integrator/1, Derivative/1, Kp/1
  Kp/1 -> Sum1/1
  Kd/1 -> Sum1/3
  Sum1/1 -> Yawrate PID/1
  Ki/1 -> Sum1/2
  Saturation/1 -> Ki/1
  Derivative/1 -> Kd/1
  Integrator/1 -> Saturation/1

== system crazyflie/On-board Controller3/Attitude Controller /Pitch PID ==
  Pitch : Inport
  Measured Pitch : Inport  Port=2
  Derivative : Derivative
  Integrator Limited : Integrator  LimitOutput=on  UpperSaturationLimit=20  LowerSaturationLimit=-20
  Kd1 : Gain  Gain=0
  Ki1 : Gain  Gain=4
  Kp1 : Gain  Gain=10
  Sum1 : Sum  Inputs=|+-
  Sum6 : Sum  Inputs=+++
  Pitch PID : Outport
  wires:
  Pitch/1 -> Sum1/1
  Measured Pitch/1 -> Sum1/2
  Sum1/1 -> Integrator Limited/1, Derivative/1, Kp1/1
  Kp1/1 -> Sum6/1
  Kd1/1 -> Sum6/3
  Sum6/1 -> Pitch PID/1
  Ki1/1 -> Sum6/2
  Derivative/1 -> Kd1/1
  Integrator Limited/1 -> Ki1/1

== system crazyflie/On-board Controller3/Attitude Controller /Roll PID ==
  Roll : Inport
  Measured Roll : Inport  Port=2
  Derivative : Derivative
  Integrator Limited : Integrator  LimitOutput=on  UpperSaturationLimit=20  LowerSaturationLimit=-20
  Kd : Gain  Gain=0
  Ki : Gain  Gain=4
  Kp : Gain  Gain=10
  Sum2 : Sum  Inputs=|+-
  Sum3 : Sum  Inputs=+++
  Roll PID : Outport
  wires:
  Roll/1 -> Sum2/1
  Measured Roll/1 -> Sum2/2
  Sum2/1 -> Integrator Limited/1, Derivative/1, Kp/1
  Kp/1 -> Sum3/1
  Kd/1 -> Sum3/3
  Sum3/1 -> Roll PID/1
  Ki/1 -> Sum3/2
  Derivative/1 -> Kd/1
  Integrator Limited/1 -> Ki/1

== system crazyflie/On-board Controller3/Attitude Rate Controller/Pitch Rate PID ==
  Pitch Ratel : Inport
  Measured Pitch Rate : Inport  Port=2
  Derivative : Derivative
  Integrator Limited : Integrator  LimitOutput=on  UpperSaturationLimit=33.3  LowerSaturationLimit=-33.3
  Kd : Gain  Gain=3
  Ki : Gain  Gain=550
  Kp : Gain  Gain=275
  Sum2 : Sum  Inputs=|+-
  Sum3 : Sum  Inputs=+++
  Pitch Rate PID : Outport
  wires:
  Pitch Ratel/1 -> Sum2/1
  Measured Pitch Rate/1 -> Sum2/2
  Sum2/1 -> Integrator Limited/1, Derivative/1, Kp/1
  Kp/1 -> Sum3/1
  Kd/1 -> Sum3/3
  Sum3/1 -> Pitch Rate PID/1
  Ki/1 -> Sum3/2
  Integrator Limited/1 -> Ki/1
  Derivative/1 -> Kd/1

== system crazyflie/On-board Controller3/Attitude Rate Controller/Roll Rate PID ==
  Roll Rate : Inport
  Measured Roll Rate : Inport  Port=2
  Derivative : Derivative
  Integrator : Integrator
  Kd : Gain  Gain=3
  Ki : Gain  Gain=550
  Kp : Gain  Gain=275
  Saturation : Saturate  UpperLimit=33.3  LowerLimit=-33.3
  Sum2 : Sum  Inputs=|+-
  Sum3 : Sum  Inputs=+++
  Roll Rate PID : Outport
  wires:
  Roll Rate/1 -> Sum2/1
  Measured Roll Rate/1 -> Sum2/2
  Sum2/1 -> Derivative/1, Integrator/1, Kp/1
  Kp/1 -> Sum3/1
  Kd/1 -> Sum3/3
  Sum3/1 -> Roll Rate PID/1
  Ki/1 -> Sum3/2
  Saturation/1 -> Ki/1
  Integrator/1 -> Saturation/1
  Derivative/1 -> Kd/1

== system crazyflie/On-board Controller3/Yawrate Controller /Yawrate PID ==
  Yawrate : Inport
  Measured Yawrate : Inport  Port=2
  Derivative : Derivative
  Integrator : Integrator
  Kd : Gain  Gain=0
  Ki : Gain  Gain=16.7
  Kp : Gain  Gain=70
  Saturation : Saturate  UpperLimit=166.7  LowerLimit=-166.7
  Sum : Sum  Inputs=|+-
  Sum1 : Sum  Inputs=+++
  Yawrate PID : Outport
  wires:
  Yawrate/1 -> Sum/1
  Measured Yawrate/1 -> Sum/2
  Sum/1 -> Integrator/1, Derivative/1, Kp/1
  Kp/1 -> Sum1/1
  Kd/1 -> Sum1/3
  Sum1/1 -> Yawrate PID/1
  Ki/1 -> Sum1/2
  Saturation/1 -> Ki/1
  Derivative/1 -> Kd/1
  Integrator/1 -> Saturation/1

== system crazyflie/On-board Controller4/Attitude Controller /Pitch PID ==
  Pitch : Inport
  Measured Pitch : Inport  Port=2
  Derivative : Derivative
  Integrator Limited : Integrator  LimitOutput=on  UpperSaturationLimit=20  LowerSaturationLimit=-20
  Kd1 : Gain  Gain=0
  Ki1 : Gain  Gain=4
  Kp1 : Gain  Gain=10
  Sum1 : Sum  Inputs=|+-
  Sum6 : Sum  Inputs=+++
  Pitch PID : Outport
  wires:
  Pitch/1 -> Sum1/1
  Measured Pitch/1 -> Sum1/2
  Sum1/1 -> Integrator Limited/1, Derivative/1, Kp1/1
  Kp1/1 -> Sum6/1
  Kd1/1 -> Sum6/3
  Sum6/1 -> Pitch PID/1
  Ki1/1 -> Sum6/2
  Derivative/1 -> Kd1/1
  Integrator Limited/1 -> Ki1/1

== system crazyflie/On-board Controller4/Attitude Controller /Roll PID ==
  Roll : Inport
  Measured Roll : Inport  Port=2
  Derivative : Derivative
  Integrator Limited : Integrator  LimitOutput=on  UpperSaturationLimit=20  LowerSaturationLimit=-20
  Kd : Gain  Gain=0
  Ki : Gain  Gain=4
  Kp : Gain  Gain=10
  Sum2 : Sum  Inputs=|+-
  Sum3 : Sum  Inputs=+++
  Roll PID : Outport
  wires:
  Roll/1 -> Sum2/1
  Measured Roll/1 -> Sum2/2
  Sum2/1 -> Integrator Limited/1, Derivative/1, Kp/1
  Kp/1 -> Sum3/1
  Kd/1 -> Sum3/3
  Sum3/1 -> Roll PID/1
  Ki/1 -> Sum3/2
  Derivative/1 -> Kd/1
  Integrator Limited/1 -> Ki/1

== system crazyflie/On-board Controller4/Attitude Rate Controller/Pitch Rate PID ==
  Pitch Ratel : Inport
  Measured Pitch Rate : Inport  Port=2
  Derivative : Derivative
  Integrator Limited : Integrator  LimitOutput=on  UpperSaturationLimit=33.3  LowerSaturationLimit=-33.3
  Kd : Gain  Gain=3
  Ki : Gain  Gain=550
  Kp : Gain  Gain=275
  Sum2 : Sum  Inputs=|+-
  Sum3 : Sum  Inputs=+++
  Pitch Rate PID : Outport
  wires:
  Pitch Ratel/1 -> Sum2/1
  Measured Pitch Rate/1 -> Sum2/2
  Sum2/1 -> Integrator Limited/1, Derivative/1, Kp/1
  Kp/1 -> Sum3/1
  Kd/1 -> Sum3/3
  Sum3/1 -> Pitch Rate PID/1
  Ki/1 -> Sum3/2
  Integrator Limited/1 -> Ki/1
  Derivative/1 -> Kd/1

== system crazyflie/On-board Controller4/Attitude Rate Controller/Roll Rate PID ==
  Roll Rate : Inport
  Measured Roll Rate : Inport  Port=2
  Derivative : Derivative
  Integrator : Integrator
  Kd : Gain  Gain=3
  Ki : Gain  Gain=550
  Kp : Gain  Gain=275
  Saturation : Saturate  UpperLimit=33.3  LowerLimit=-33.3
  Sum2 : Sum  Inputs=|+-
  Sum3 : Sum  Inputs=+++
  Roll Rate PID : Outport
  wires:
  Roll Rate/1 -> Sum2/1
  Measured Roll Rate/1 -> Sum2/2
  Sum2/1 -> Derivative/1, Integrator/1, Kp/1
  Kp/1 -> Sum3/1
  Kd/1 -> Sum3/3
  Sum3/1 -> Roll Rate PID/1
  Ki/1 -> Sum3/2
  Saturation/1 -> Ki/1
  Integrator/1 -> Saturation/1
  Derivative/1 -> Kd/1

== system crazyflie/On-board Controller4/Yawrate Controller /Yawrate PID ==
  Yawrate : Inport
  Measured Yawrate : Inport  Port=2
  Derivative : Derivative
  Integrator : Integrator
  Kd : Gain  Gain=0
  Ki : Gain  Gain=16.7
  Kp : Gain  Gain=70
  Saturation : Saturate  UpperLimit=166.7  LowerLimit=-166.7
  Sum : Sum  Inputs=|+-
  Sum1 : Sum  Inputs=+++
  Yawrate PID : Outport
  wires:
  Yawrate/1 -> Sum/1
  Measured Yawrate/1 -> Sum/2
  Sum/1 -> Integrator/1, Derivative/1, Kp/1
  Kp/1 -> Sum1/1
  Kd/1 -> Sum1/3
  Sum1/1 -> Yawrate PID/1
  Ki/1 -> Sum1/2
  Saturation/1 -> Ki/1
  Derivative/1 -> Kd/1
  Integrator/1 -> Saturation/1

== matlab function crazyflie/Dynamics/Angular Acceleration ==
  data: F1 input double [0..1]; pqr_dot_x output; F2 input double [0..1]; F3 input double [0..1]; F4 input double [0..1]; M1 input; M2 input; M3 input; M4 input; pqr input
function pqr_dot_x = Crazyflie_ang(F1,F2,F3,F4,M1,M2,M3,M4,pqr)
%#codegen
pqr_dot_x = zeros(3,1);
L = 0.0455;
Ixx = 2.3951E-05;
Iyy = 2.3951E-05;
Izz = 3.2347E-05;
I_matrix = diag([Ixx Iyy Izz]);

Eq1 = [L/sqrt(2)*(F3+F4-F1-F2); ...
      L/sqrt(2)*(F1+F4-F2-F3); ...
      -M1+M2-M3+M4];
Eq2 = cross(pqr, I_matrix*pqr);
  
pqr_dot = inv(I_matrix)*(Eq1 - Eq2);


pqr_dot_x = pqr_dot;

== matlab function crazyflie/Dynamics/Acceleration ==
  data: F1 input double; F2 input; F3 input; F4 input; r_dot_dot output; rpy input
function r_dot_dot = Crazyflie_accel(F1,F2,F3,F4,rpy)
%#codegen
r_dot_dot = zeros(3,1);
m = 0.041;
g = [0;0;-9.81];

Wrb = [cos(rpy(3))*cos(rpy(2))+sin(rpy(1))*sin(rpy(2))*sin(rpy(3)) -cos(rpy(1))*sin(rpy(3)) cos(rpy(3))*sin(rpy(2))-cos(rpy(2))*sin(rpy(1))*sin(rpy(3)); ...
       cos(rpy(2))*sin(rpy(3))-cos(rpy(3))*sin(rpy(1))*sin(rpy(2)) cos(rpy(1))*cos(rpy(3)) sin(rpy(3))*sin(rpy(2))+cos(rpy(3))*cos(rpy(2))*sin(rpy(1)); ...
       -cos(rpy(1))*sin(rpy(2)) -sin(rpy(1)) cos(rpy(1))*cos(rpy(2))];  
r_dot_dot = g + 1/m * Wrb*[0;0;sum([F1 F2 F3 F4])];

== matlab function crazyflie/Dynamics/Acceleration1 ==
  data: pqr input; rpy_dot output; rpy input
function rpy_dot = Crazyflie_rpy(pqr, rpy)
%#codegen
rpy_dot = zeros(3,1);
Wrb = [cos(rpy(2)) 0 -cos(rpy(1))*sin(rpy(2)); ...
       0 1 sin(rpy(1)); ...
       sin(rpy(2)) 0 cos(rpy(1))*cos(rpy(2))];
  
rpy_dot = Wrb\pqr;

== matlab function crazyflie/Off-board PID Position Controller/Subsystem/MATLAB Function ==
  data: yaw input; R_m output
function R_m = Error_transform(yaw)
%#codegen

R_m = [cos(yaw) sin(yaw); -sin(yaw) cos(yaw)];

== matlab function crazyflie/Off-board PID Position Controller1/Subsystem/MATLAB Function ==
  data: yaw input; R_m output
function R_m = Error_transform(yaw)
%#codegen

R_m = eye(2);
%[cos(yaw) sin(yaw); -sin(yaw) cos(yaw)];

== matlab function crazyflie/Dynamics1/Acceleration ==
  data: F1 input double; F2 input; F3 input; F4 input; r_dot_dot output; rpy input
function r_dot_dot = Crazyflie_accel(F1,F2,F3,F4,rpy)
%#codegen
r_dot_dot = zeros(3,1);
m = 0.041;
g = [0;0;-9.81];

Wrb = [cos(rpy(3))*cos(rpy(2))+sin(rpy(1))*sin(rpy(2))*sin(rpy(3)) -cos(rpy(1))*sin(rpy(3)) cos(rpy(3))*sin(rpy(2))-cos(rpy(2))*sin(rpy(1))*sin(rpy(3)); ...
       cos(rpy(2))*sin(rpy(3))-cos(rpy(3))*sin(rpy(1))*sin(rpy(2)) cos(rpy(1))*cos(rpy(3)) sin(rpy(3))*sin(rpy(2))+cos(rpy(3))*cos(rpy(2))*sin(rpy(1)); ...
       -cos(rpy(1))*sin(rpy(2)) -sin(rpy(1)) cos(rpy(1))*cos(rpy(2))];  
r_dot_dot = g + 1/m * Wrb*[0;0;sum([F1 F2 F3 F4])];

== matlab function crazyflie/Dynamics1/Acceleration1 ==
  data: pqr input; rpy_dot output; rpy input
function rpy_dot = Crazyflie_rpy(pqr, rpy)
%#codegen
rpy_dot = zeros(3,1);
Wrb = [cos(rpy(2)) 0 -cos(rpy(1))*sin(rpy(2)); ...
       0 1 sin(rpy(1)); ...
       sin(rpy(2)) 0 cos(rpy(1))*cos(rpy(2))];
  
rpy_dot = Wrb\pqr;

== matlab function crazyflie/Dynamics1/Angular Acceleration ==
  data: F1 input double [0..1]; pqr_dot_x output; F2 input double [0..1]; F3 input double [0..1]; F4 input double [0..1]; M1 input; M2 input; M3 input; M4 input; pqr input
function pqr_dot_x = Crazyflie_ang(F1,F2,F3,F4,M1,M2,M3,M4,pqr)
%#codegen
pqr_dot_x = zeros(3,1);
L = 0.0455;
Ixx = 2.3951E-05;
Iyy = 2.3951E-05;
Izz = 3.2347E-05;
I_matrix = diag([Ixx Iyy Izz]);

Eq1 = [L/sqrt(2)*(F3+F4-F1-F2); ...
      L/sqrt(2)*(F1+F4-F2-F3); ...
      -M1+M2-M3+M4];
Eq2 = cross(pqr, I_matrix*pqr);
  
pqr_dot = inv(I_matrix)*(Eq1 - Eq2);


pqr_dot_x = pqr_dot;

== matlab function crazyflie/Off-board LQR Position Controller /Subsystem/MATLAB Function ==
  data: yaw input; R_m output
function R_m = Error_transform(yaw)
%#codegen

R_m = [cos(yaw) sin(yaw); -sin(yaw) cos(yaw)];

== matlab function crazyflie/Dynamics2/Acceleration ==
  data: F1 input double; F2 input; F3 input; F4 input; r_dot_dot output; rpy input
function r_dot_dot = Crazyflie_accel(F1,F2,F3,F4,rpy)
%#codegen
r_dot_dot = zeros(3,1);
m = 0.041;
g = [0;0;-9.81];

Wrb = [cos(rpy(3))*cos(rpy(2))+sin(rpy(1))*sin(rpy(2))*sin(rpy(3)) -cos(rpy(1))*sin(rpy(3)) cos(rpy(3))*sin(rpy(2))-cos(rpy(2))*sin(rpy(1))*sin(rpy(3)); ...
       cos(rpy(2))*sin(rpy(3))-cos(rpy(3))*sin(rpy(1))*sin(rpy(2)) cos(rpy(1))*cos(rpy(3)) sin(rpy(3))*sin(rpy(2))+cos(rpy(3))*cos(rpy(2))*sin(rpy(1)); ...
       -cos(rpy(1))*sin(rpy(2)) -sin(rpy(1)) cos(rpy(1))*cos(rpy(2))];  
r_dot_dot = g + 1/m * Wrb*[0;0;sum([F1 F2 F3 F4])];

== matlab function crazyflie/Dynamics2/Acceleration1 ==
  data: pqr input; rpy_dot output; rpy input
function rpy_dot = Crazyflie_rpy(pqr, rpy)
%#codegen
rpy_dot = zeros(3,1);
Wrb = [cos(rpy(2)) 0 -cos(rpy(1))*sin(rpy(2)); ...
       0 1 sin(rpy(1)); ...
       sin(rpy(2)) 0 cos(rpy(1))*cos(rpy(2))];
  
rpy_dot = Wrb\pqr;

== matlab function crazyflie/Dynamics2/Angular Acceleration ==
  data: F1 input double [0..1]; pqr_dot_x output; F2 input double [0..1]; F3 input double [0..1]; F4 input double [0..1]; M1 input; M2 input; M3 input; M4 input; pqr input
function pqr_dot_x = Crazyflie_ang(F1,F2,F3,F4,M1,M2,M3,M4,pqr)
%#codegen
pqr_dot_x = zeros(3,1);
L = 0.0455;
Ixx = 2.3951E-05;
Iyy = 2.3951E-05;
Izz = 3.2347E-05;
I_matrix = diag([Ixx Iyy Izz]);

Eq1 = [L/sqrt(2)*(F3+F4-F1-F2); ...
      L/sqrt(2)*(F1+F4-F2-F3); ...
      -M1+M2-M3+M4];
Eq2 = cross(pqr, I_matrix*pqr);
  
pqr_dot = inv(I_matrix)*(Eq1 - Eq2);


pqr_dot_x = pqr_dot;
